simulink model "Ex3_2_4_old"  (R2022b)
settings: Solver=VariableStepAuto  StartTime=0.0  StopTime=30  RelTol=1e-3
settings Model: Creator=15043  LastModifiedBy=15043

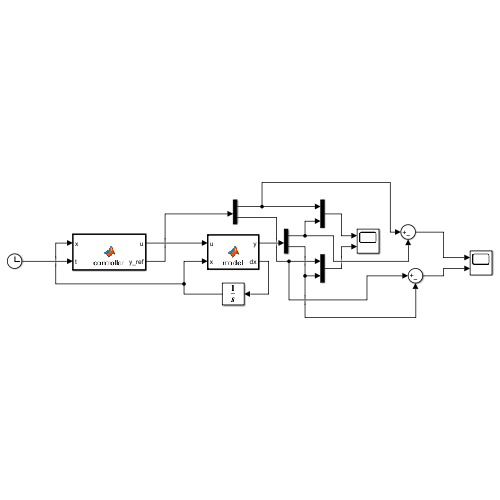
[thumbnail: Simulink's stored preview of the top-level diagram]
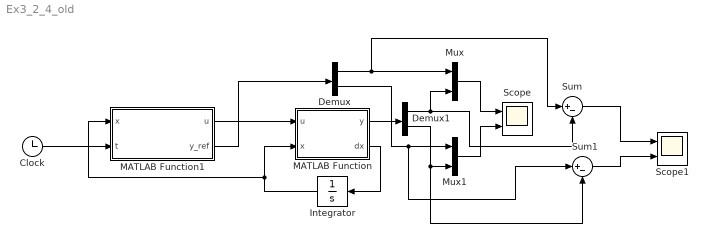
== system Ex3_2_4_old ==
  Clock : Clock
  Demux : Demux  Outputs=2
  Demux1 : Demux  Outputs=2
  Integrator : Integrator  InitialCondition=[0;0;0;0;0;]
  MATLAB Function : MATLAB Function  TreatAsAtomicUnit=on
  MATLAB Function1 : MATLAB Function  TreatAsAtomicUnit=on
  Mux : Mux  Inputs=2
  Mux1 : Mux  Inputs=2
  Scope : Scope  NumInputPorts=2
  Scope1 : Scope  NumInputPorts=2
  Sum : Sum  Inputs=|+-
  Sum1 : Sum  Inputs=|+-
  wires:
  MATLAB Function/2(dx) -> Integrator/1
  Integrator/1 -> MATLAB Function1/1(x), MATLAB Function/2(x)
  MATLAB Function/1(y) -> Demux1/1
  Demux/1 -> Sum/1, Mux/1
  Demux1/1 -> Mux/2, Sum/2
  Mux/1 -> Scope/1
  Mux1/1 -> Scope/2
  Demux1/2 -> Mux1/2, Sum1/2
  Demux/2 -> Sum1/1, Mux1/1
  Sum1/1 -> Scope1/2
  Sum/1 -> Scope1/1
  MATLAB Function1/1(u) -> MATLAB Function/1(u)
  MATLAB Function1/2(y_ref) -> Demux/1
  Clock/1 -> MATLAB Function1/2(t)

== matlab function Ex3_2_4_old/MATLAB Function1 ==
  data: x input; u output; t input; y_ref output
function [u, y_ref]  = controller(x,t)
    y10 = 0;
    y20 = 0;
    y1T = 2;
    y2T = 3;
    T = 10;
    
    y1_ref = (3*t^2/T^2 - 2*t^3/T^3)*(y1T - y10)+ y10;
    y2_ref = (3*t^2/T^2 - 2*t^3/T^3)*(y2T - y20)+ y20;
    y_ref = [y1_ref; y2_ref;];
    y_ref_dot = [3*t/25 - 3*t^2/250; 9*t/50 - 9*t^2/500];
    
    v = [-0.1*(x(3)-y_ref(1)); -0.1*(x(2)-y_ref(2))]; % introduced new input of the linearized system
    u = ([x(1)-x(3);-x(1)*x(3)-x(4)] +y_ref_dot + v); % control law
end

== matlab function Ex3_2_4_old/MATLAB Function ==
  data: u input; y output; x input; dx output
function [y, dx] = model(u, x)
    x1 = x(1);
    x2 = x(2);
    x3 = x(3);
    x4 = x(4);
    x5 = x(5);
    
    f = [ -x1 + x2^2;
           x1*x3 + x4;
          -x1 + x3;
           x5;
          -x5 + x3^2;];
    g = [ 0 0; 0 1; 1 0; 1 0; x2 0;];
    dx = f + g*u;

    y = [x3; x2;];
end
